simulink model "Quad_PID_controller"  (R2016a)
settings: Solver=ode45  StartTime=0.0  StopTime=40  RelTol=1e-3
InitFcn:
  | kTau = 1.63
  | l = 0.23
  | pul_force = 1.22061*9.8/1000
  | slope=0.576
  | motorMass = 0.1
  | armMass = 0.07
  | upperLimitOfCalibration = 1600
  | lowerLimitOfCalibration = 1000
  | g = 9.81
undefined symbols (not defined in the file or in its folder): LowerLimitOfCalibration, UpperLimitOfCalibration
libraries: simulink x1
settings Model: Creator=Nikhil  LastModifiedBy=manoj
settings DataIOCC: LimitDataPoints=on  SaveFormat=Array
settings DebuggingCC: SolverPrmCheckMsg=warning
settings HardwareCC: ProdBitPerPointer=32  ProdLargestAtomicFloat=None  ProdIntDivRoundTo=Undefined  ProdEndianess=Unspecified  ProdWordSize=32  ProdHWDeviceType=32-bit Generic
settings ModelReferenceCC: PropagateSignalLabelsOutOfModel=off
settings ConfigComp: CovModelRefEnable=Off  CovSFcnEnable=off
settings ConfigurationSet: Description=SimMechanics 2G

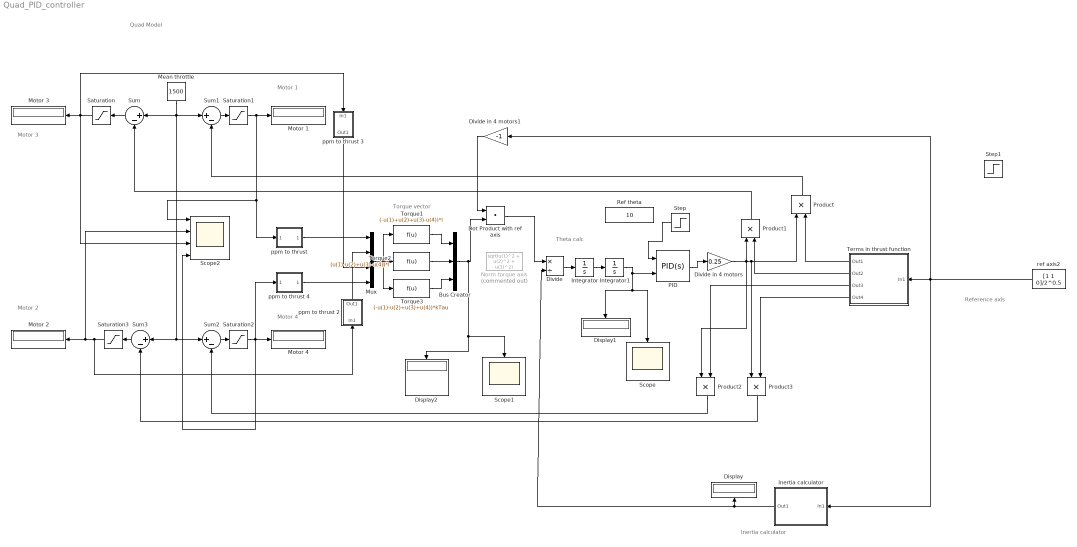
== system Quad_PID_controller ==
  note: Torque vector
  note: Reference axis
  note: Quad Model
  note: Motor 1
  note: Motor 2
  note: Motor 4
  note: Motor 3
  note: Inertia calculator
  note: Theta calc
  Bus Creator : BusCreator  Inputs=3
  Display : Display
  Display1 : Display
  Display2 : Display
  Divide : Product  Inputs=*/
  Divide in 4 motors : Gain  Gain=0.25
  Divide in 4 motors1 : Gain  Gain=-1
  Dot Product with ref axis : DotProduct  InputSameDT=on  OutDataTypeStr=Inherit: Inherit via internal rule
  Inertia calculator : Subsystem
  Integrator : Integrator
  Integrator1 : Integrator
  Mean throttle : Constant  Value=1500
  Motor {1..4} (4 alike) : Display
  Mux : Mux
  Norm torque axis : Fcn  Commented=on  Expr=sqrt(u(1)^2 + u(2)^2 + u(3)^2)
  PID : simulink/Continuous/PID Controller (2DOF)  Controller=PID  TimeDomain=Continuous-time  SampleTime=-1  IntegratorMethod=Forward Euler  FilterMethod=Forward Euler  Form=Parallel  UseFilter=on  ControllerParametersSource=internal  P=250  I=50  D=39.6424116843145  N=27.269851271081  b=0.921263095055131  c=0.714061468846318  InitialConditionSource=internal  InitialConditionForIntegrator=0  InitialConditionForFilter=0  ExternalReset=none  LimitOutput=off  UpperSaturationLimit=inf  LowerSaturationLimit=-inf  LinearizeAsGain=on  AntiWindupMode=none  Kb=1  TrackingMode=off  Kt=1  PParamMin=[]  PParamMax=[]  IParamMin=[]  IParamMax=[]  DParamMin=[]  DParamMax=[]  NParamMin=[]  NParamMax=[]  bParamMin=[]  bParamMax=[]  cParamMin=[]  cParamMax=[]  KbParamMin=[]  KbParamMax=[]  KtParamMin=[]  KtParamMax=[]  POutMin=[]  POutMax=[]  IOutMin=[]  IOutMax=[]  DOutMin=[]  DOutMax=[]  NOutMin=[]  NOutMax=[]  bOutMin=[]  bOutMax=[]  cOutMin=[]  cOutMax=[]  KbOutMin=[]  KbOutMax=[]  KtOutMin=[]  KtOutMax=[]  IntegratorOutMin=[]  IntegratorOutMax=[]  FilterOutMin=[]  FilterOutMax=[]  SumOutMin=[]  SumOutMax=[]  Sum1OutMin=[]  Sum1OutMax=[]  Sum2OutMin=[]  Sum2OutMax=[]  Sum3OutMin=[]  Sum3OutMax=[]  SumI1OutMin=[]  SumI1OutMax=[]  SumI2OutMin=[]  SumI2OutMax=[]  SumI3OutMin=[]  SumI3OutMax=[]  SumDOutMin=[]  SumDOutMax=[]  SaturationOutMin=[]  SaturationOutMax=[]  IntegratorContinuousStateAttributes=''  IntegratorStateMustResolveToSignalObject=off  IntegratorRTWStateStorageClass=Auto  FilterContinuousStateAttributes=''  FilterStateMustResolveToSignalObject=off  FilterRTWStateStorageClass=Auto  DifferentiatorICPrevScaledInput=0  DifferentiatorOutMin=[]  DifferentiatorOutMax=[]
  Product{,1..3} (4 alike) : Product
  Ref theta : Constant  Value=10
  Saturation{,1..3} (4 alike) : Saturate  UpperLimit=upperLimitOfCalibration  LowerLimit=lowerLimitOfCalibration
  Scope : Scope
  Scope1 : Scope
  Scope2 : Scope  NumInputPorts=4
  Step : Step  Time=20  Before=10  After=0  SampleTime=0
  Step1 : Step  Time=40  Before=[0 0 1]  After=[1 0 0]  SampleTime=0  VectorParams1D=off
  Sum{,1..3} (4 alike) : Sum  Inputs=|+-
  Terms in thrust function : Subsystem
  Torque1 : Fcn  Expr=(-u(1)+u(2)+u(3)-u(4))*l
  Torque2 : Fcn  Expr=(u(1)-u(2)+u(3)-u(4))*l
  Torque3 : Fcn  Expr=(-u(1)-u(2)+u(3)+u(4))*kTau
  ppm to thrust : Subsystem
  ppm to thrust 2 : Subsystem
  ppm to thrust 3 : Subsystem
  ppm to thrust 4 : Subsystem
  ref axis2 : Constant  Value=[1 1 0]/2^0.5
  wires:
  Sum1/1 -> Saturation1/1
  Sum3/1 -> Saturation3/1
  Mux/1 -> Torque3/1, Torque2/1, Torque1/1
  ppm to thrust/1(Out1) -> Mux/1
  ppm to thrust 4/1(Out1) -> Mux/4
  ppm to thrust 2/1(Out1) -> Mux/2
  ppm to thrust 3/1(Out1) -> Mux/3
  Sum2/1 -> Saturation2/1
  PID/1 -> Divide in 4 motors/1
  Divide in 4 motors/1 -> Product1/1, Product/1, Product3/1, Product2/1
  Product/1 -> Sum1/2
  Product1/1 -> Sum/2
  Product2/1 -> Sum2/2
  Product3/1 -> Sum3/2
  Torque1/1 -> Bus Creator/1
  Torque2/1 -> Bus Creator/2
  Divide/1 -> Integrator/1
  Integrator/1 -> Integrator1/1
  Integrator1/1 -> PID/2, Scope/1, Display1/1
  Inertia calculator/1(Out1) -> Divide/2, Display/1
  Terms in thrust function/1(Out1) -> Product/2
  Terms in thrust function/2(Out2) -> Product1/2
  Terms in thrust function/3(Out3) -> Product2/2
  Terms in thrust function/4(Out4) -> Product3/2
  Mean throttle/1 -> Sum1/1, Sum/1, Sum2/1, Sum3/1
  Sum/1 -> Saturation/1
  Saturation/1 -> Scope2/3, ppm to thrust 3/1(In1), Motor 3/1
  Saturation1/1 -> Scope2/1, ppm to thrust/1(In1), Motor 1/1
  Saturation3/1 -> ppm to thrust 2/1(In1), Scope2/2, Motor 2/1
  ref axis2/1 -> Divide in 4 motors1/1, Inertia calculator/1(In1), Terms in thrust function/1(In1)
  Divide in 4 motors1/1 -> Dot Product with ref axis/1
  Dot Product with ref axis/1 -> Divide/1
  Torque3/1 -> Bus Creator/3
  Bus Creator/1 -> Dot Product with ref axis/2, Scope1/1, Display2/1
  Saturation2/1 -> Scope2/4, ppm to thrust 4/1(In1), Motor 4/1
  Step/1 -> PID/1

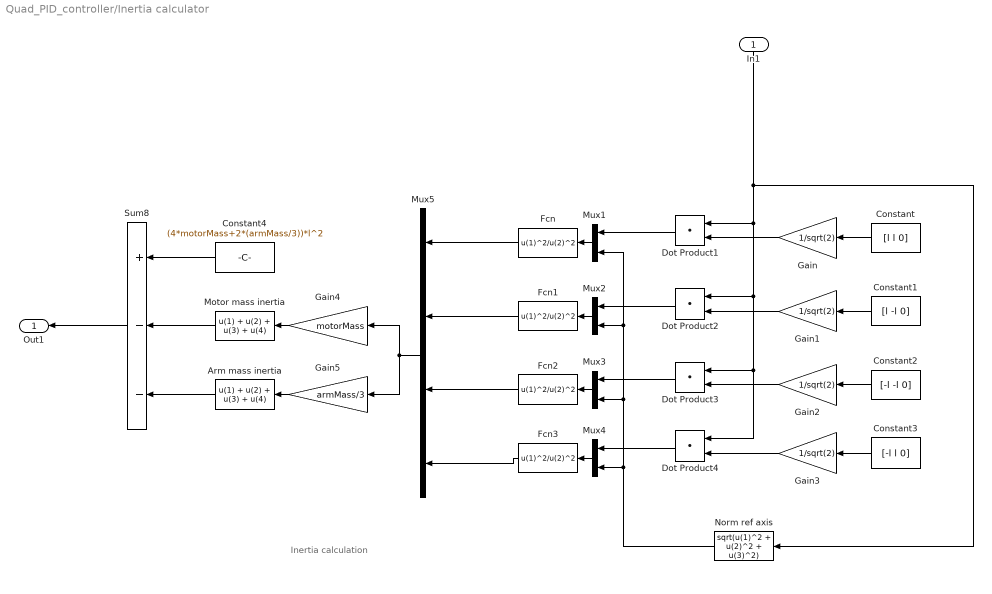
== system Quad_PID_controller/Inertia calculator ==
  note: Inertia calculation
  In1 : Inport
  Arm mass inertia : Fcn  Expr=u(1) + u(2) + u(3) + u(4)
  Constant : Constant  Value=[l l 0]
  Constant1 : Constant  Value=[l -l 0]
  Constant2 : Constant  Value=[-l -l 0]
  Constant3 : Constant  Value=[-l l 0]
  Constant4 : Constant  Value=(4*motorMass+2*(armMass/3))*l^2
  Dot Product1 : DotProduct  InputSameDT=on  OutDataTypeStr=Inherit: Inherit via internal rule
  Dot Product2 : DotProduct  InputSameDT=on  OutDataTypeStr=Inherit: Inherit via internal rule
  Dot Product3 : DotProduct  InputSameDT=on  OutDataTypeStr=Inherit: Inherit via internal rule
  "Dot Product4 " : DotProduct  InputSameDT=on  OutDataTypeStr=Inherit: Inherit via internal rule
  Fcn{,1..3} (4 alike) : Fcn  Expr=u(1)^2/u(2)^2
  Gain{,1..3} (4 alike) : Gain  Gain=1/sqrt(2)
  Gain4 : Gain  Gain=motorMass
  Gain5 : Gain  Gain=armMass/3
  Motor mass inertia : Fcn  Expr=u(1) + u(2) + u(3) + u(4)
  Mux{1..4} (4 alike) : Mux  Inputs=2
  Mux5 : Mux
  Norm ref axis : Fcn  Expr=sqrt(u(1)^2 + u(2)^2 + u(3)^2)
  Sum8 : Sum  Inputs=+--
  Out1 : Outport
  wires:
  Sum8/1 -> Out1/1
  Constant4/1 -> Sum8/1
  Constant2/1 -> Gain2/1
  Mux3/1 -> Fcn2/1
  Gain/1 -> Dot Product1/2
  Constant3/1 -> Gain3/1
  Gain2/1 -> Dot Product3/2
  Dot Product1/1 -> Mux1/1
  Gain1/1 -> Dot Product2/2
  Mux1/1 -> Fcn/1
  Constant/1 -> Gain/1
  Mux2/1 -> Fcn1/1
  Gain3/1 -> "Dot Product4 "/2
  "Dot Product4 "/1 -> Mux4/1
  Constant1/1 -> Gain1/1
  Mux4/1 -> Fcn3/1
  Norm ref axis/1 -> Mux4/2, Mux3/2, Mux2/2, Mux1/2
  Dot Product2/1 -> Mux2/1
  Dot Product3/1 -> Mux3/1
  Fcn/1 -> Mux5/1
  Mux5/1 -> Gain4/1, Gain5/1
  Fcn3/1 -> Mux5/4
  Motor mass inertia/1 -> Sum8/2
  Fcn2/1 -> Mux5/3
  Gain4/1 -> Motor mass inertia/1
  Arm mass inertia/1 -> Sum8/3
  Gain5/1 -> Arm mass inertia/1
  Fcn1/1 -> Mux5/2
  In1/1 -> Norm ref axis/1, "Dot Product4 "/1, Dot Product3/1, Dot Product2/1, Dot Product1/1

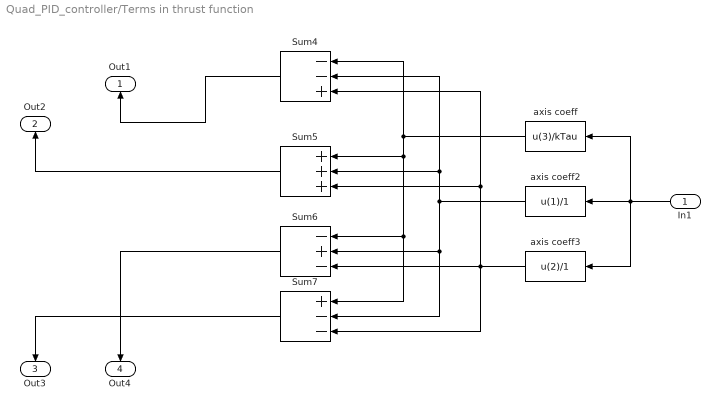
== system Quad_PID_controller/Terms in thrust function ==
  In1 : Inport
  Sum4 : Sum  Inputs=--+
  Sum5 : Sum  Inputs=+++
  Sum6 : Sum  Inputs=-+-
  Sum7 : Sum  Inputs=+--
  axis coeff : Fcn  Expr=u(3)/kTau
  axis coeff2 : Fcn  Expr=u(1)/1
  axis coeff3 : Fcn  Expr=u(2)/1
  Out1 : Outport
  Out2 : Outport  Port=2
  Out3 : Outport  Port=3
  Out4 : Outport  Port=4
  wires:
  axis coeff/1 -> Sum4/1, Sum7/1, Sum6/1, Sum5/1
  axis coeff3/1 -> Sum6/3, Sum7/3, Sum4/3, Sum5/3
  axis coeff2/1 -> Sum4/2, Sum5/2, Sum7/2, Sum6/2
  Sum7/1 -> Out3/1
  Sum5/1 -> Out2/1
  Sum6/1 -> Out4/1
  Sum4/1 -> Out1/1
  In1/1 -> axis coeff3/1, axis coeff2/1, axis coeff/1

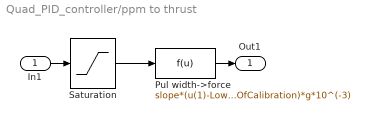
== system Quad_PID_controller/ppm to thrust ==
  In1 : Inport
  Pul width->force : Fcn  Expr=slope*(u(1)-LowerLimitOfCalibration)*g*10^(-3)
  Saturation : Saturate  UpperLimit=UpperLimitOfCalibration  LowerLimit=LowerLimitOfCalibration
  Out1 : Outport
  wires:
  Pul width->force/1 -> Out1/1
  In1/1 -> Saturation/1
  Saturation/1 -> Pul width->force/1

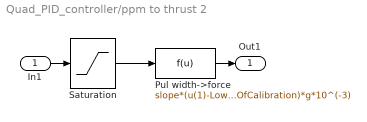
== system Quad_PID_controller/ppm to thrust 2 ==
  In1 : Inport
  Pul width->force : Fcn  Expr=slope*(u(1)-LowerLimitOfCalibration)*g*10^(-3)
  Saturation : Saturate  UpperLimit=UpperLimitOfCalibration  LowerLimit=LowerLimitOfCalibration
  Out1 : Outport
  wires:
  Pul width->force/1 -> Out1/1
  In1/1 -> Saturation/1
  Saturation/1 -> Pul width->force/1

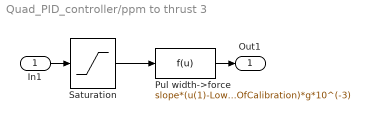
== system Quad_PID_controller/ppm to thrust 3 ==
  In1 : Inport
  Pul width->force : Fcn  Expr=slope*(u(1)-LowerLimitOfCalibration)*g*10^(-3)
  Saturation : Saturate  UpperLimit=UpperLimitOfCalibration  LowerLimit=LowerLimitOfCalibration
  Out1 : Outport
  wires:
  Saturation/1 -> Pul width->force/1
  In1/1 -> Saturation/1
  Pul width->force/1 -> Out1/1

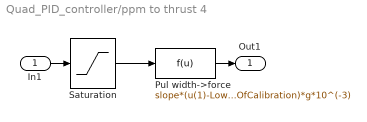
== system Quad_PID_controller/ppm to thrust 4 ==
  In1 : Inport
  Pul width->force : Fcn  Expr=slope*(u(1)-LowerLimitOfCalibration)*g*10^(-3)
  Saturation : Saturate  UpperLimit=UpperLimitOfCalibration  LowerLimit=LowerLimitOfCalibration
  Out1 : Outport
  wires:
  Saturation/1 -> Pul width->force/1
  In1/1 -> Saturation/1
  Pul width->force/1 -> Out1/1
